simulink model "sineinput1_closedloop_simulation"  (R2023a)
settings: Solver=VariableStepAuto  StartTime=0.0  StopTime=10.0  RelTol=1e-3
settings Model: Creator=anshu  LastModifiedBy=anshu

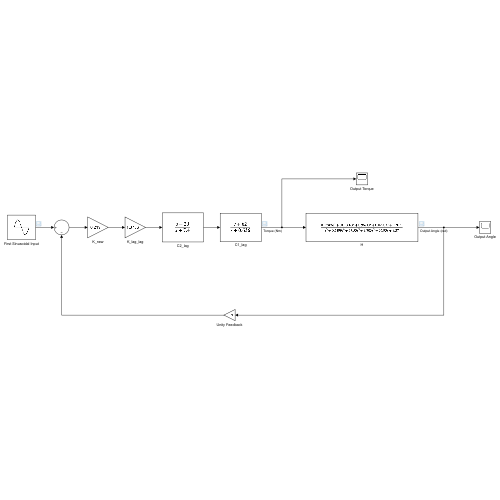
[thumbnail: Simulink's stored preview of the top-level diagram]
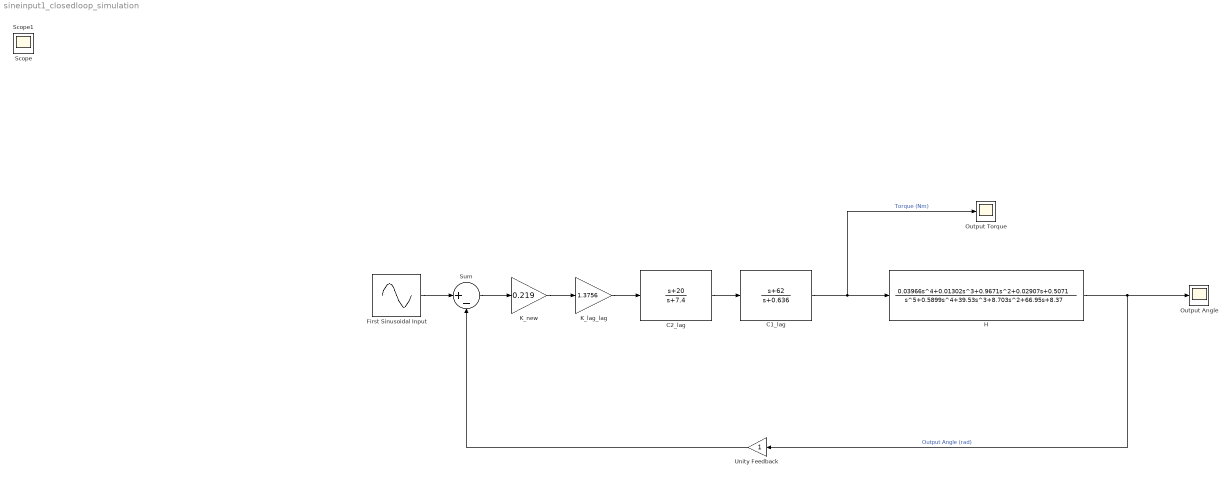
== system sineinput1_closedloop_simulation ==
  C1_lag : TransferFcn  Numerator=[1 62]  Denominator=[1 0.636]
  C2_lag : TransferFcn  Numerator=[1 20]  Denominator=[1 7.4]
  First Sinusoidal Input : Sin  Amplitude=0.5  Frequency=3.14  SampleTime=0
  H : TransferFcn  Numerator=[0.03966 0.01302 0.9671 0.02907 0.5071]  Denominator=[1 0.5899 39.53 8.703 66.95 8.37]
  K_lag_lag : Gain  Gain=1.3756
  K_new : Gain  Gain=0.219
  Output Angle : Scope
  Output Torque : Scope
  Sum : Sum  Inputs=|+-
  Unity Feedback : Gain
  Scope : Scope
  Scope1 : Scope
  wires:
  First Sinusoidal Input/1 -> Sum/1
  K_lag_lag/1 -> C2_lag/1
  K_new/1 -> K_lag_lag/1
  H/1 -> Unity Feedback/1, Output Angle/1  "Output Angle (rad)"
  Unity Feedback/1 -> Sum/2
  C2_lag/1 -> C1_lag/1
  Sum/1 -> K_new/1
  C1_lag/1 -> Output Torque/1, H/1  "Torque (Nm)"
